simulink model "pi_controller"  (R2024a)
settings: Solver=ode15s  StartTime=0.0  StopTime=10.0  RelTol=1e-3
model mask{ki=7.33, kp=9.39, ts=.01}
  mask prompts: ki "integral gain"; kp "proportional gain"; ts "sample time"
model workspace (MAT data in the model file):
  ki = 7.33
  kp = 9.39
  ts = 0.01
  v = 7.4
settings Model: ParameterArgumentNames=ki,kp,ts  Creator=awabm  LastModifiedBy=awabm
settings DataIOCC: SaveOutput=off  SaveTime=off

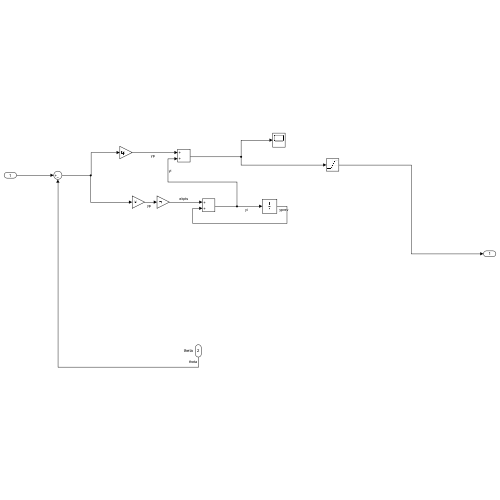
[thumbnail: Simulink's stored preview of the top-level diagram]
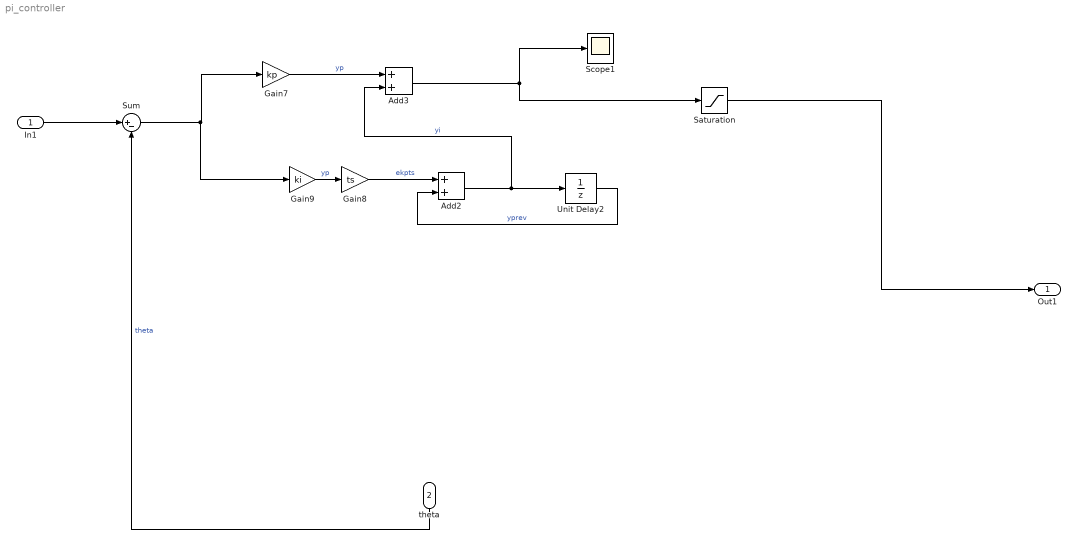
== system pi_controller ==
  In1 : Inport  OutDataTypeStr=double  PortDimensions=1
  theta : Inport  Port=2  OutDataTypeStr=double  PortDimensions=1  SampleTime=0
  Add2 : Sum
  Add3 : Sum
  Gain7 : Gain  Gain=kp
  Gain8 : Gain  Gain=ts
  Gain9 : Gain  Gain=ki
  Saturation : Saturate  UpperLimit=v  LowerLimit=-v
  Scope1 : Scope
  Sum : Sum  Inputs=|+-
  Unit Delay2 : UnitDelay  SampleTime=ts  HasFrameUpgradeWarning=on
  Out1 : Outport  OutDataTypeStr=double  PortDimensions=1  SampleTime=0
  wires:
  Add2/1 -> Unit Delay2/1, Add3/2  "yi"
  Unit Delay2/1 -> Add2/2  "yprev"
  Gain7/1 -> Add3/1  "yp"
  Gain8/1 -> Add2/1  "ekpts"
  Sum/1 -> Gain7/1, Gain9/1
  Add3/1 -> Scope1/1, Saturation/1
  Saturation/1 -> Out1/1
  Gain9/1 -> Gain8/1  "yp"
  theta/1 -> Sum/2  "theta"
  In1/1 -> Sum/1
